simulink model "pendule_inv_echant_etu"  (R2017a)
settings: Solver=VariableStepAuto  StartTime=0.0  StopTime=10.0  RelTol=1e-3
values from neighbouring files (symbols this model uses):
  delta_t = 0.4    [exemple_test_pendule_inv_echant.m]
  K = [10 1]    [exemple_test_pendule_inv_capteur.m]    (also in exemple_test_pendule_inv_echant.m = [30 10])
  ue = 0    [exemple_test_pendule_inv_capteur.m]    (also in exemple_test_pendule_inv_echant.m)
  x0 = [pi/20 0]    [exemple_test_pendule_inv_capteur.m]    (also in exemple_test_pendule_inv_echant.m)
  xe = [0 0]    [exemple_test_pendule_inv_capteur.m]    (also in exemple_test_pendule_inv_echant.m)
undefined symbols (not defined in the file or in its folder): DiscIntNeverNeededParam
settings Model: Creator=jky  LastModifiedBy=jky

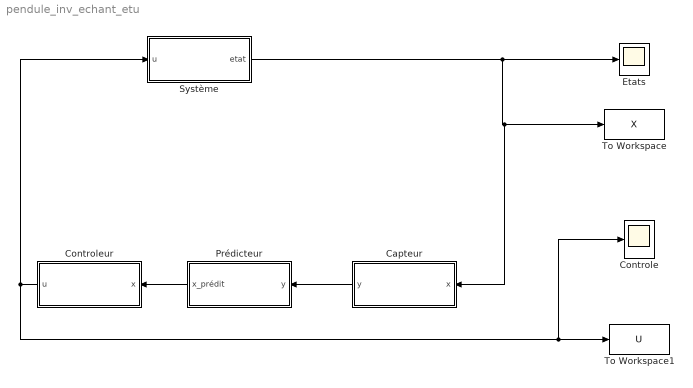
== system pendule_inv_echant_etu ==
  Capteur : Subsystem
  Controle : Scope
  Controleur : Subsystem
  Etats : Scope
  Prédicteur : Subsystem
  Système : Subsystem
  To Workspace : ToWorkspace  VariableName=X  SaveFormat=Timeseries  SampleTime=-1
  To Workspace1 : ToWorkspace  VariableName=U  SaveFormat=Timeseries  SampleTime=-1
  wires:
  Prédicteur/1("x_prédit ") -> Controleur/1(x)
  Controleur/1(u) -> Système/1(u), Controle/1, To Workspace1/1
  Capteur/1(y) -> Prédicteur/1(y)
  Système/1(etat) -> Capteur/1(x), To Workspace/1, Etats/1

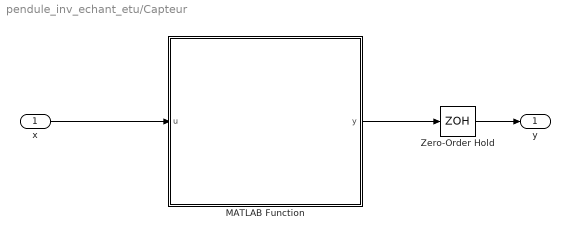
== system pendule_inv_echant_etu/Capteur ==
  x : Inport
  MATLAB Function : MATLAB Function  TreatAsAtomicUnit=on
  Zero-Order Hold : ZeroOrderHold  SampleTime=delta_t
  y : Outport
  wires:
  MATLAB Function/1(y) -> Zero-Order Hold/1
  x/1 -> MATLAB Function/1(u)
  Zero-Order Hold/1 -> y/1

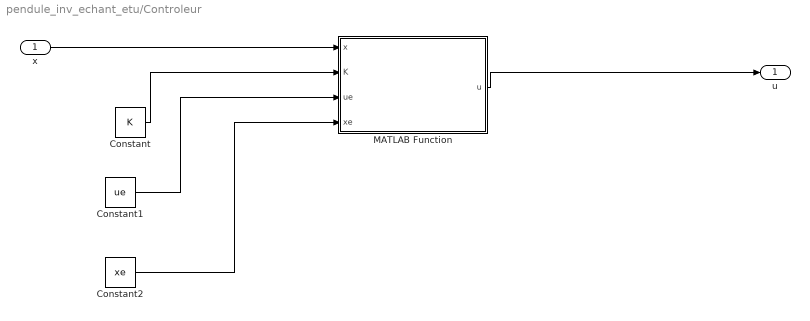
== system pendule_inv_echant_etu/Controleur ==
  x : Inport
  Constant : Constant  Value=K
  Constant1 : Constant  Value=ue
  Constant2 : Constant  Value=xe
  MATLAB Function : MATLAB Function  TreatAsAtomicUnit=on
  u : Outport
  wires:
  x/1 -> MATLAB Function/1(x)
  MATLAB Function/1(u) -> u/1
  Constant/1 -> MATLAB Function/2(K)
  Constant1/1 -> MATLAB Function/3(ue)
  Constant2/1 -> MATLAB Function/4(xe)

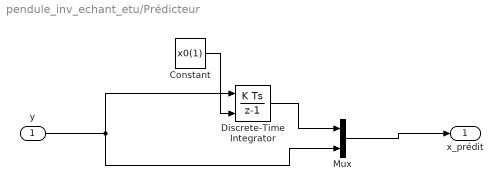
== system pendule_inv_echant_etu/Prédicteur ==
  y : Inport
  Constant : Constant  Value=x0(1)
  Discrete-Time Integrator : DiscreteIntegrator  InitialConditionSource=external  InitialConditionSetting=State (most efficient)  SampleTime=-1  ICPrevOutput=DiscIntNeverNeededParam  ICPrevScaledInput=DiscIntNeverNeededParam
  Mux : Mux  Inputs=2
  "x_prédit " : Outport
  wires:
  Discrete-Time Integrator/1 -> Mux/1
  Mux/1 -> "x_prédit "/1
  y/1 -> Mux/2, Discrete-Time Integrator/1
  Constant/1 -> Discrete-Time Integrator/2

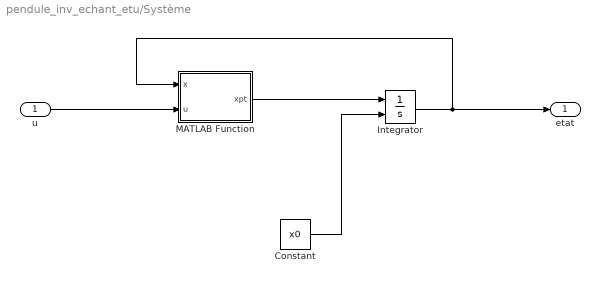
== system pendule_inv_echant_etu/Système ==
  u : Inport
  Constant : Constant  Value=x0
  Integrator : Integrator  InitialConditionSource=external  InitialCondition=[pi/20 0]
  MATLAB Function : MATLAB Function  TreatAsAtomicUnit=on
  etat : Outport
  wires:
  Constant/1 -> Integrator/2
  u/1 -> MATLAB Function/2(u)
  Integrator/1 -> etat/1, MATLAB Function/1(x)
  MATLAB Function/1(xpt) -> Integrator/1

== matlab function pendule_inv_echant_etu/Controleur/MATLAB Function ==
  data: x input; u output; K input; ue input; xe input
function u = fcn(x, K, ue, xe)
u = ue + K(:)'*(x(:)-xe);

== matlab function pendule_inv_echant_etu/Système/MATLAB Function ==
  data: x input; u input; xpt output
function xpt = fcn(x,u)
g = 9.81;
l = 10;
xpt = transpose([x(2) ((g/l)*sin(x(1)))-((cos(x(1))*u)/l)]);

== matlab function pendule_inv_echant_etu/Capteur/MATLAB Function ==
  data: u input; y output
function y = fcn(u)

y = u(2);
